simulink model "suspension_sys_ex3"  (Simulink 7.0)
settings: Solver=ode23t  StartTime=0.0  StopTime=10.0  RelTol=1e-3
libraries: fl_lib x14, nesl_utility x8
settings Model: Creator=kiran.jacob  LastModifiedBy=kiran.jacob

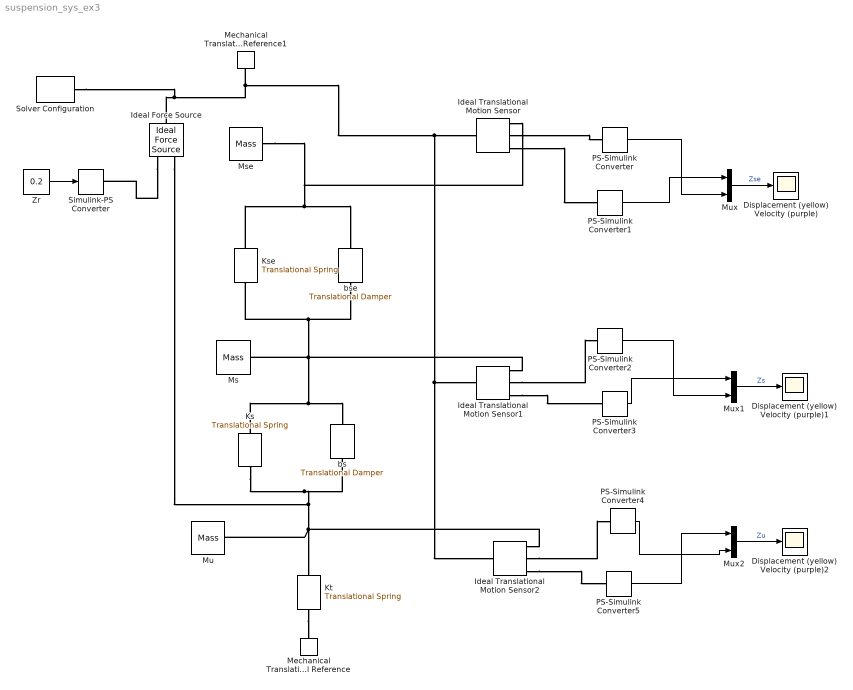
== system suspension_sys_ex3 ==
  " Ks" : fl_lib/Mechanical/Translational Elements/Translational Spring  Orientation=down  DialogController=NetworkEngine.DynNeDlgSource  SystemSampleTime=-1  spr_rate=28000 N/m  init_def=0 m  force_Log=off  deformation_Log=off  LocalVarNames=|force|deformation  LocalVarDescs=|Spring force (N)|Spring deformation (m)  LocalVarLogging=[0 0]
  " Kse" : fl_lib/Mechanical/Translational Elements/Translational Spring  Orientation=down  DialogController=NetworkEngine.DynNeDlgSource  SystemSampleTime=-1  spr_rate=8000 N/m  init_def=0 m  force_Log=off  deformation_Log=off  LocalVarNames=|force|deformation  LocalVarDescs=|Spring force (N)|Spring deformation (m)  LocalVarLogging=[0 0]
  " Kt" : fl_lib/Mechanical/Translational Elements/Translational Spring  Orientation=down  DialogController=NetworkEngine.DynNeDlgSource  SystemSampleTime=-1  spr_rate=125000 N/m  init_def=0 m  force_Log=off  deformation_Log=off  LocalVarNames=|force|deformation  LocalVarDescs=|Spring force (N)|Spring deformation (m)  LocalVarLogging=[0 0]
  Displacement (yellow) Velocity (purple) : Scope
      settings: TimeRange=10  YMin=-6e-006  YMax=1.2e-005  SaveName=ScopeData6
  Displacement (yellow) Velocity (purple)1 : Scope
      settings: TimeRange=10  YMin=-6e-006  YMax=1.4e-005
  Displacement (yellow) Velocity (purple)2 : Scope
      settings: TimeRange=10  YMin=-9.999999999999999e-006  YMax=6e-005
  Ideal Force Source : fl_lib/Mechanical/Mechanical Sensors and Sources/Ideal Force Source  Orientation=down  DialogController=NetworkEngine.DynNeDlgSource  SystemSampleTime=-1  force_Log=off  rel_velocity_Log=off  power_Log=off  LocalVarNames=|force|rel_velocity|power  LocalVarDescs=|Force (N)|Relative velocity (m/s)|Power generated by the source (W)  LocalVarLogging=[0 0 0]
  Ideal Translational Motion Sensor : fl_lib/Mechanical/Mechanical Sensors and Sources/Ideal Translational Motion Sensor  DialogController=NetworkEngine.DynNeDlgSource  SystemSampleTime=-1  offset=0 m  LocalVarLogging=[]
  Ideal Translational Motion Sensor1 : fl_lib/Mechanical/Mechanical Sensors and Sources/Ideal Translational Motion Sensor  DialogController=NetworkEngine.DynNeDlgSource  SystemSampleTime=-1  offset=0 m  LocalVarLogging=[]
  Ideal Translational Motion Sensor2 : fl_lib/Mechanical/Mechanical Sensors and Sources/Ideal Translational Motion Sensor  DialogController=NetworkEngine.DynNeDlgSource  SystemSampleTime=-1  offset=0 m  LocalVarLogging=[]
  Mechanical Translational Reference : fl_lib/Mechanical/Translational Elements/Mechanical Translational Reference  Orientation=down  DialogController=NetworkEngine.DynNeDlgSource  SystemSampleTime=-1  LocalVarLogging=[]
  Mechanical Translational Reference1 : fl_lib/Mechanical/Translational Elements/Mechanical Translational Reference  Orientation=up  DialogController=NetworkEngine.DynNeDlgSource  SystemSampleTime=-1  LocalVarLogging=[]
  Ms : fl_lib/Mechanical/Translational Elements/Mass  Orientation=left  DialogController=NetworkEngine.DynNeDlgSource  SystemSampleTime=-1  mass=250 kg  initial_velocity=0 m/s  force_Log=off  velocity_Log=off  LocalVarNames=|force|velocity  LocalVarDescs=|Inertia force (N)|Mass absolute velocity (m/s)  LocalVarLogging=[0 0]
  Mse : fl_lib/Mechanical/Translational Elements/Mass  Orientation=left  DialogController=NetworkEngine.DynNeDlgSource  SystemSampleTime=-1  mass=90 kg  initial_velocity=0 m/s  force_Log=off  velocity_Log=off  LocalVarNames=|force|velocity  LocalVarDescs=|Inertia force (N)|Mass absolute velocity (m/s)  LocalVarLogging=[0 0]
  Mu : fl_lib/Mechanical/Translational Elements/Mass  Orientation=left  DialogController=NetworkEngine.DynNeDlgSource  SystemSampleTime=-1  mass=40 kg  initial_velocity=0 m/s  force_Log=off  velocity_Log=off  LocalVarNames=|force|velocity  LocalVarDescs=|Inertia force (N)|Mass absolute velocity (m/s)  LocalVarLogging=[0 0]
  Mux : Mux  Inputs=2
  Mux1 : Mux  Inputs=2
  Mux2 : Mux  Inputs=2
  PS-Simulink Converter{,1..5} (6 alike) : nesl_utility/PS-Simulink Converter  DialogController=NetworkEngine.DynNeUtilDlgSource  SystemSampleTime=-1  PhysicalDomain=network_engine_domain  LeftPortType=input  RightPortType=output  SubClassName=ps_output  Unit=1
  Simulink-PS Converter : nesl_utility/Simulink-PS Converter  DialogController=NetworkEngine.DynNeUtilDlgSource  SystemSampleTime=-1  PhysicalDomain=network_engine_domain  LeftPortType=input  RightPortType=output  SubClassName=ps_input  Unit=1
  Solver Configuration : nesl_utility/Solver Configuration  DialogController=NetworkEngine.DynNeUtilDlgSource  SystemSampleTime=-1  PhysicalDomain=network_engine_domain  LeftPortType=input  RightPortType=generic  SubClassName=solver  ResidualTolerance=1e-9  MaxNonlinIter=12  MaxModeIter=2  DoFixedCost=off  DoDC=off  LinearAlgebra=Sparse  Accelerate=off
  Zr : Constant  Value=0.2  OutDataType=sfix(16)  OutScaling=2^0
  bs : fl_lib/Mechanical/Translational Elements/Translational Damper  Orientation=down  DialogController=NetworkEngine.DynNeDlgSource  SystemSampleTime=-1  D=2000 N/(m/s)  force_Log=off  rel_velocity_Log=off  power_Log=off  LocalVarNames=|force|rel_velocity|power  LocalVarDescs=|Damping force (N)|Damper relative velocity (m/s)|Power dissipated in the damper (W)  LocalVarLogging=[0 0 0]
  bse : fl_lib/Mechanical/Translational Elements/Translational Damper  Orientation=down  DialogController=NetworkEngine.DynNeDlgSource  SystemSampleTime=-1  D=3000 N/(m/s)  force_Log=off  rel_velocity_Log=off  power_Log=off  LocalVarNames=|force|rel_velocity|power  LocalVarDescs=|Damping force (N)|Damper relative velocity (m/s)|Power dissipated in the damper (W)  LocalVarLogging=[0 0 0]
  wires:
  Zr/1 -> Simulink-PS Converter/1
  Mux/1 -> Displacement (yellow) Velocity (purple)/1  "Zse"
  Mux1/1 -> Displacement (yellow) Velocity (purple)1/1  "Zs"
  Mux2/1 -> Displacement (yellow) Velocity (purple)2/1  "Zu"
  PS-Simulink Converter3/1 -> Mux1/1
  PS-Simulink Converter2/1 -> Mux1/2
  PS-Simulink Converter1/1 -> Mux/1
  PS-Simulink Converter/1 -> Mux/2
  PS-Simulink Converter5/1 -> Mux2/1
  PS-Simulink Converter4/1 -> Mux2/2
  connections:
  " Kse"/RConn1 -- bse/RConn1 -- " Ks"/LConn1 -- bs/LConn1 -- Ms/LConn1 -- Ideal Translational Motion Sensor1/RConn1
  Ideal Translational Motion Sensor/RConn2 -- PS-Simulink Converter/LConn1
  Ideal Translational Motion Sensor/RConn3 -- PS-Simulink Converter1/LConn1
  " Ks"/RConn1 -- bs/RConn1 -- " Kt"/LConn1 -- Mu/LConn1 -- Ideal Translational Motion Sensor2/RConn1 -- Ideal Force Source/RConn2
  Ideal Translational Motion Sensor1/RConn3 -- PS-Simulink Converter3/LConn1
  Ideal Translational Motion Sensor1/RConn2 -- PS-Simulink Converter2/LConn1
  " Kt"/RConn1 -- Mechanical Translational Reference/LConn1
  Ideal Force Source/RConn1 -- Simulink-PS Converter/RConn1
  Ideal Translational Motion Sensor2/RConn2 -- PS-Simulink Converter4/LConn1
  Ideal Translational Motion Sensor2/RConn3 -- PS-Simulink Converter5/LConn1
  Mse/LConn1 -- bse/LConn1 -- " Kse"/LConn1 -- Ideal Translational Motion Sensor/RConn1
  Ideal Force Source/LConn1 -- Solver Configuration/RConn1 -- Mechanical Translational Reference1/LConn1 -- Ideal Translational Motion Sensor/LConn1 -- Ideal Translational Motion Sensor1/LConn1 -- Ideal Translational Motion Sensor2/LConn1
